simulink model "Project_part3"  (R2024b)
settings: Solver=VariableStepAuto  StartTime=0.0  StopTime=0.05  RelTol=1e-3
values from neighbouring files (symbols this model uses):
  fs = 1000    [part2 - overshootandsettlingtime.m]    (also in projectpart5.m)
  Hc = (1/Hf) * (Ho/(1-Ho))    [projectpart5.m]
  Hf = tf(sys)    [projectpart5.m]
settings Model: Creator=Talida  LastModifiedBy=Talida

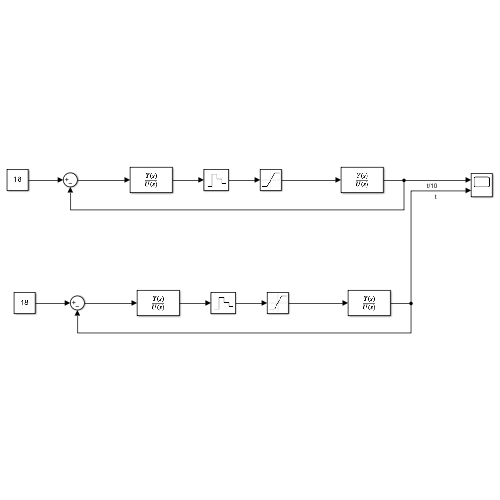
[thumbnail: Simulink's stored preview of the top-level diagram]
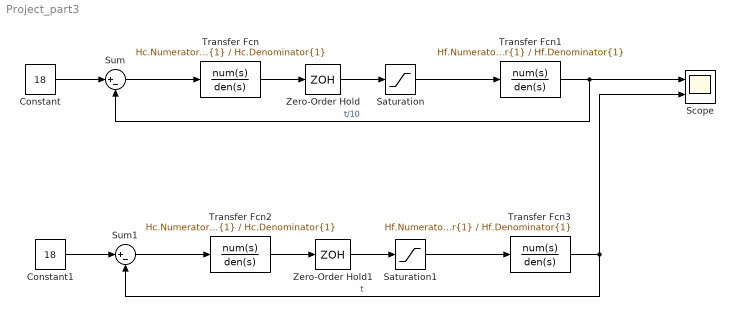
== system Project_part3 ==
  Constant : Constant  Value=18
  Constant1 : Constant  Value=18
  Saturation : Saturate  UpperLimit=1  LowerLimit=0
  Saturation1 : Saturate  UpperLimit=1  LowerLimit=0
  Scope : Scope  NumInputPorts=2
  Sum : Sum  Inputs=|+-
  Sum1 : Sum  Inputs=|+-
  Transfer Fcn : TransferFcn  Numerator=Hc.Numerator{1}  Denominator=Hc.Denominator{1}
  Transfer Fcn1 : TransferFcn  Numerator=Hf.Numerator{1}  Denominator=Hf.Denominator{1}
  Transfer Fcn2 : TransferFcn  Numerator=Hc.Numerator{1}  Denominator=Hc.Denominator{1}
  Transfer Fcn3 : TransferFcn  Numerator=Hf.Numerator{1}  Denominator=Hf.Denominator{1}
  Zero-Order Hold : ZeroOrderHold  SampleTime=1/fs/10
  Zero-Order Hold1 : ZeroOrderHold  SampleTime=1/fs
  wires:
  Constant/1 -> Sum/1
  Sum/1 -> Transfer Fcn/1
  Transfer Fcn/1 -> Zero-Order Hold/1
  Zero-Order Hold/1 -> Saturation/1
  Saturation/1 -> Transfer Fcn1/1
  Transfer Fcn1/1 -> Sum/2, Scope/1  "t/10"
  Zero-Order Hold1/1 -> Saturation1/1
  Sum1/1 -> Transfer Fcn2/1
  Transfer Fcn3/1 -> Scope/2, Sum1/2  "t"
  Constant1/1 -> Sum1/1
  Transfer Fcn2/1 -> Zero-Order Hold1/1
  Saturation1/1 -> Transfer Fcn3/1
